simulink model "mars_landing"  (R2016b)
settings: Solver=FixedStepDiscrete  StartTime=0.0  StopTime=750  FixedStep=0.1  RelTol=1e-3
PostLoadFcn:
  | init_model
values from neighbouring files (symbols this model uses):
  InitialHeight = 10000    [calibration.mat]
  InitialVelocity = 0    [calibration.mat]
settings Model: Creator=csax  LastModifiedBy=csax
settings OptimizationCC: DefaultParameterBehavior=Inlined
settings DebuggingCC: ParameterTunabilityLossMsg=error
settings HardwareCC: ProdBitPerPointer=32  ProdBitPerSizeT=32  ProdBitPerPtrDiffT=32  ProdLargestAtomicFloat=None  ProdWordSize=32  ProdHWDeviceType=Custom Processor->Custom
settings RTWCC: SystemTargetFile=trace32_target_ert.tlc  MakeCommand=trace32_target_make  TemplateMakefile=trace32_arm_tmf.tmf  Description=TRACE32 Target
settings CodeAppCC: ForceParamTrailComments=on  IgnoreCustomStorageClasses=off  OperatorAnnotations=on  SimulinkDataObjDesc=on  SFDataObjDesc=on  MATLABFcnDesc=on  InsertBlockDesc=on  MATLABSourceComments=on
settings STFCustomTargetCC: TargetLangStandard=C99 (ISO)  CombineOutputUpdateFcns=on  ERTCustomFileBanners=on  SupportContinuousTime=off  SupportNonInlinedSFcns=off  RemoveResetFunc=on  MATLABClassNameForMDSCustomization=Simulink.SoftwareTarget.ERTCustomization  GRTInterface=off  SystemTargetFile=trace32_target_ert.tlc
settings ERTTargetCC: TargetLangStandard=C99 (ISO)  ParMdlRefBuildCompliant=off  CompOptLevelCompliant=off  ConcurrentExecutionCompliant=off  ERTFirstTimeCompliant=off  ModelStepFunctionPrototypeControlCompliant=off  CPPClassGenCompliant=off  UseToolchainInfoCompliant=off  InlinedParameterPlacement=NonHierarchical  ERTCustomFileTemplate=example_file_process.tlc

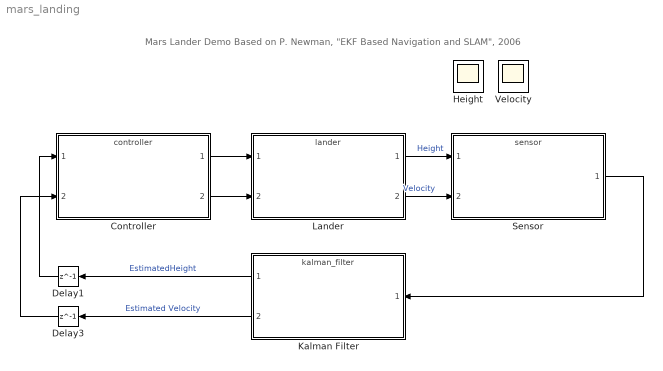
== system mars_landing ==
  note: Mars Lander Demo
      |
      | Based on P. Newman, "EKF Based Navigation and SLAM", 2006
  Controller : ModelReference  ModelNameDialog=controller.slx  SimulationMode=Normal  ModelReferenceVersion=1.40
  Delay1 : Delay  DelayLength=1  InitialCondition=InitialHeight
  Delay3 : Delay  DelayLength=1  InitialCondition=InitialVelocity
  Height : Scope
      settings: Floating=on
  Kalman Filter : ModelReference  ModelNameDialog=kalman_filter.slx  SimulationMode=Processor-in-the-loop (PIL)  ModelReferenceVersion=1.102
  Lander : ModelReference  ModelNameDialog=lander.slx  SimulationMode=Normal  ModelReferenceVersion=1.86
  Sensor : ModelReference  ModelNameDialog=sensor.slx  SimulationMode=Normal  ModelReferenceVersion=1.26
  Velocity : Scope
      settings: Floating=on
  wires:
  Lander/1 -> Sensor/1  "Height"
  Lander/2 -> Sensor/2  "Velocity"
  Sensor/1 -> Kalman Filter/1
  Controller/1 -> Lander/1
  Controller/2 -> Lander/2
  Kalman Filter/1 -> Delay1/1  "EstimatedHeight"
  Kalman Filter/2 -> Delay3/1  "Estimated Velocity"
  Delay3/1 -> Controller/2
  Delay1/1 -> Controller/1
